simulink model "WindTunnelControl"  (R2023b)
settings: Solver=FixedStepDiscrete  StartTime=0.0  StopTime=Config.simulationTime  FixedStep=Config.tStep  RelTol=1e-3
InitFcn:
  | cd(fileparts(which(bdroot)));
  | initWindTunnelControl;
  | 
  | %% Try to edit the GUI (the user may have already closed it)
  | try
  | 
  |     %% Update Start Button
  |     set(sl_synch_handles.startButton,'Backgroundcolor',[0.0,1.0,0.0]);
  |     set(sl_synch_handles.startButton,'Enable','on');
  | end
StartFcn:
  | %% Try to edit the GUI (the user may have already closed it)
  | try
  | 
  |     %% Update Start Button
  |     set(sl_synch_handles.startButton,'Backgroundcolor',[0.8,0.8,0.8]);
  |     set(sl_synch_handles.startButton,'Enable','off');
  | 
  |     %% Update Compile Button
  |     set(sl_synch_handles.compileButton,'Backgroundcolor',[0.8,0.8,0.8]);
  |     set(sl_synch_handles.compileButton,'Enable','off');
  | 
  |     %% Update Exit Button
  |     set(sl_synch_handles.exitButton,'Backgroundcolor',[0.8,0.8,0.8]);
  |     set(sl_synch_handles.exitButton,'Enable','off');
  | end
StopFcn:
  | cd(fileparts(which(bdroot)));
  | stopWindTunnelControl;
  | 
  | %% Try to edit the GUI (the user may have already closed it)
  | try
  | 
  |     %% Update Start Button
  |     if get(sl_synch_handles.checkbox_recompile, 'Value')
  |         set(sl_synch_handles.startButton,'Backgroundcolor',[0.0,1.0,0.0]);
  |         set(sl_synch_handles.startButton,'Enable','on');
  |     end
  | 
  |     %% Update Compile Button
  |     set(sl_synch_handles.compileButton,'Backgroundcolor',[1.0,0.6,0.0]);
  |     set(sl_synch_handles.compileButton,'Enable','on');
  | 
  |     %% Update Exit Button
  |     set(sl_synch_handles.exitButton,'Backgroundcolor',[0.0,1.0,1.0]);
  |     set(sl_synch_handles.exitButton,'Enable','on');
  | end
undefined symbols (not defined in the file or in its folder): Config
libraries: dspsigattribs x44, WBToolboxLibrary x37, Get_System_State x1, Dynamics_and_Kinematics x1
CloseFcn:
  | %% Try to close the GUI (the user might have already closed it)
  | try
  | 
  |     close(simulinkStaticGUI)
  | end
settings Model: NumberOfSteps=50  Creator=gnava  LastModifiedBy=icub
settings SolverCC: AlgebraicLoopSolver=TrustRegion
settings DataIOCC: ReturnWorkspaceOutputs=off
settings OptimizationCC: BlockReduction=off  DefaultParameterBehavior=Inlined  BufferReuse=off  ReuseModelBlockBuffer=off
settings DebuggingCC: UnconnectedInputMsg=warning  UnconnectedOutputMsg=warning  UnconnectedLineMsg=warning  ArithmeticOperatorsInVariantConditions=warning
settings ModelReferenceCC: EnableRefExpFcnMdlSchedulingChecks=on
settings SFSimCC: SimUseLocalCustomCode=off  CustomCodeUndefinedFunction=UseInterfaceOnly
settings RTWCC: RTWUseLocalCustomCode=off  DLArmComputeVersion=19.05

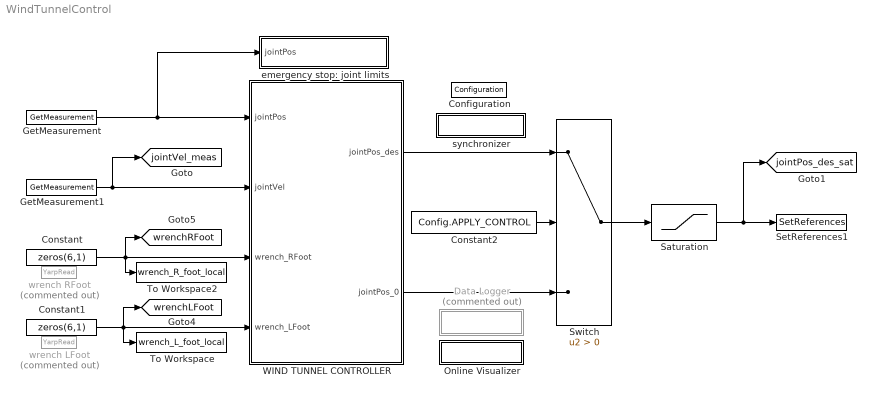
== system WindTunnelControl ==
  Configuration : WBToolboxLibrary/Utilities/Configuration  ConfigSource=Workspace  ConfigObject='WBTConfigRobot'
      settings: SourceProductName=WholeBodyToolbox
  Constant : Constant  Value=zeros(6,1)
  Constant1 : Constant  Value=zeros(6,1)
  Constant2 : Constant  Value=Config.APPLY_CONTROL  VectorParams1D=off  SampleTime=-1
  Data Logger : Subsystem  Commented=on
      mask Display: disp('DATA LOGGER')
  GetMeasurement : WBToolboxLibrary/States/GetMeasurement  measuredType=Joints Position
      settings: SourceProductName=WholeBodyToolbox
  GetMeasurement1 : WBToolboxLibrary/States/GetMeasurement  measuredType=Joints Velocity
      settings: SourceProductName=WholeBodyToolbox
  Online Visualizer : Subsystem
      mask Display: disp('VISUALIZER')
  Saturation : Saturate  UpperLimit=Config.sat.jointPositionLimits(:,2)  LowerLimit=Config.sat.jointPositionLimits(:,1)
  SetReferences1 : WBToolboxLibrary/Actuators/SetReferences  controlType=Position Direct  refSpeed=10*(pi/180)  refAcceleration=1000000*(pi/180)
      settings: SourceProductName=WholeBodyToolbox
  Switch : Switch  Criteria=u2 > Threshold  SaturateOnIntegerOverflow=off  InputSameDT=off
  To Workspace : ToWorkspace  VariableName=wrench_L_foot_local  SaveFormat=Structure With Time  SampleTime=-1
  To Workspace2 : ToWorkspace  VariableName=wrench_R_foot_local  SaveFormat=Structure With Time  SampleTime=-1
  WIND TUNNEL CONTROLLER : Subsystem
  emergency stop: joint limits : Subsystem
      mask Display: disp('EMERGENCY STOP')
  synchronizer : Subsystem
      mask Display: disp('SYNCHRONIZER')
  wrench LFoot : WBToolboxLibrary/Utilities/YarpRead  Commented=on  portName=Ports.WRENCH_LEFT_FOOT  signalSize=6  timeout=0.5  blocking=off  timestamp=off  autoconnect=on  errorOnConnection=on
      settings: SourceProductName=WholeBodyToolbox
  wrench RFoot : WBToolboxLibrary/Utilities/YarpRead  Commented=on  portName=Ports.WRENCH_RIGHT_FOOT  signalSize=6  timeout=0.5  blocking=off  timestamp=off  autoconnect=on  errorOnConnection=on
      settings: SourceProductName=WholeBodyToolbox
  tag scope: jointPos_des_sat=global, jointVel_meas=global, wrenchLFoot=global, wrenchRFoot=global
  wires:
  GetMeasurement1/1 -> [jointVel_meas], WIND TUNNEL CONTROLLER/2(jointVel)
  GetMeasurement/1 -> emergency stop: joint limits/1(jointPos), WIND TUNNEL CONTROLLER/1(jointPos)
  Constant2/1 -> Switch/2
  WIND TUNNEL CONTROLLER/1(jointPos_des) -> Switch/1
  Switch/1 -> Saturation/1
  WIND TUNNEL CONTROLLER/2(jointPos_0) -> Switch/3
  Saturation/1 -> [jointPos_des_sat], SetReferences1/1
  Constant1/1 -> [wrenchLFoot], To Workspace/1, WIND TUNNEL CONTROLLER/4(wrench_LFoot)
  Constant/1 -> To Workspace2/1, [wrenchRFoot], WIND TUNNEL CONTROLLER/3(wrench_RFoot)

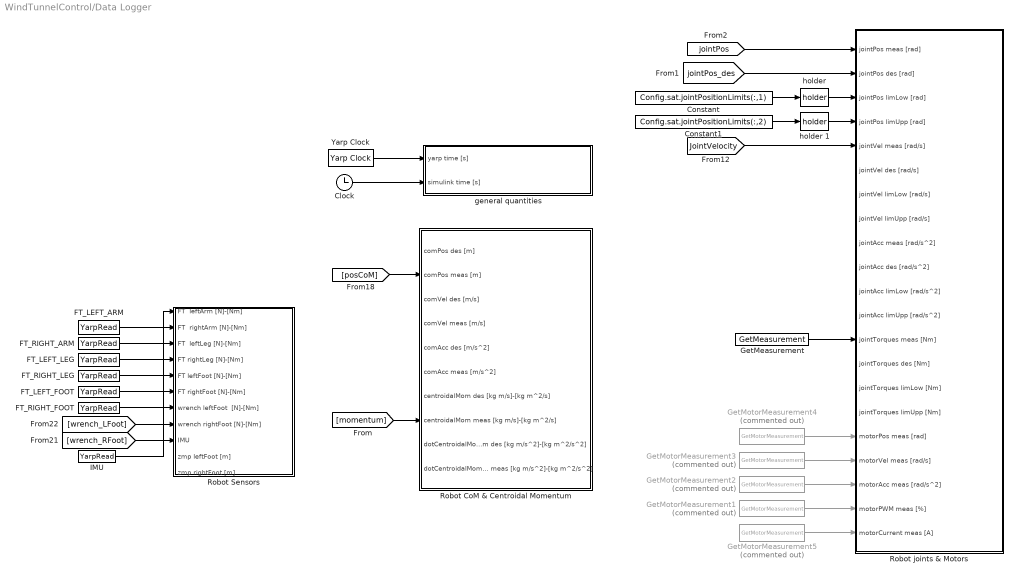
== system WindTunnelControl/Data Logger ==
  Clock : Clock
  Constant : Constant  Value=Config.sat.jointPositionLimits(:,1)
  Constant1 : Constant  Value=Config.sat.jointPositionLimits(:,2)
  FT_LEFT_ARM : WBToolboxLibrary/Utilities/YarpRead  portName=Ports.FT_LEFT_ARM  signalSize=6  timeout=0.5  blocking=off  timestamp=off  autoconnect=on  errorOnConnection=on
      settings: SourceProductName=WholeBodyToolbox
  FT_LEFT_FOOT : WBToolboxLibrary/Utilities/YarpRead  portName=Ports.FT_LEFT_FOOT  signalSize=6  timeout=0.5  blocking=off  timestamp=off  autoconnect=on  errorOnConnection=on
      settings: SourceProductName=WholeBodyToolbox
  FT_LEFT_LEG : WBToolboxLibrary/Utilities/YarpRead  portName=Ports.FT_LEFT_LEG  signalSize=6  timeout=0.5  blocking=off  timestamp=off  autoconnect=on  errorOnConnection=on
      settings: SourceProductName=WholeBodyToolbox
  FT_RIGHT_ARM : WBToolboxLibrary/Utilities/YarpRead  portName=Ports.FT_RIGHT_ARM  signalSize=6  timeout=0.5  blocking=off  timestamp=off  autoconnect=on  errorOnConnection=on
      settings: SourceProductName=WholeBodyToolbox
  FT_RIGHT_FOOT : WBToolboxLibrary/Utilities/YarpRead  portName=Ports.FT_RIGHT_FOOT  signalSize=6  timeout=0.5  blocking=off  timestamp=off  autoconnect=on  errorOnConnection=on
      settings: SourceProductName=WholeBodyToolbox
  FT_RIGHT_LEG : WBToolboxLibrary/Utilities/YarpRead  portName=Ports.FT_RIGHT_LEG  signalSize=6  timeout=0.5  blocking=off  timestamp=off  autoconnect=on  errorOnConnection=on
      settings: SourceProductName=WholeBodyToolbox
  GetMeasurement : WBToolboxLibrary/States/GetMeasurement  measuredType=Joints Torque
      settings: SourceProductName=WholeBodyToolbox
  GetMotorMeasurement1 : WBToolboxLibrary/States/GetMotorMeasurement  Commented=on  measuredType=Motor PWM
      settings: SourceProductName=WholeBodyToolbox
  GetMotorMeasurement2 : WBToolboxLibrary/States/GetMotorMeasurement  Commented=on  measuredType=Motor Acceleration
      settings: SourceProductName=WholeBodyToolbox
  GetMotorMeasurement3 : WBToolboxLibrary/States/GetMotorMeasurement  Commented=on  measuredType=Motor Velocity
      settings: SourceProductName=WholeBodyToolbox
  GetMotorMeasurement4 : WBToolboxLibrary/States/GetMotorMeasurement  Commented=on  measuredType=Motor Position
      settings: SourceProductName=WholeBodyToolbox
  GetMotorMeasurement5 : WBToolboxLibrary/States/GetMotorMeasurement  Commented=on  measuredType=Motor Current
      settings: SourceProductName=WholeBodyToolbox
  IMU : WBToolboxLibrary/Utilities/YarpRead  portName=Ports.IMU  signalSize=12  timeout=0.5  blocking=off  timestamp=off  autoconnect=on  errorOnConnection=on
      settings: SourceProductName=WholeBodyToolbox
  Robot CoM & Centroidal Momentum : Subsystem  AncestorBlock=data_dumper/Robot CoM & Centroidal Momentum
      settings: LibrarySourceBlock=data_dumper/Robot CoM & Centroidal Momentum
  Robot Sensors : Subsystem  AncestorBlock=data_dumper/Robot Sensors
      settings: LibrarySourceBlock=data_dumper/Robot Sensors
  Robot joints & Motors : Subsystem  AncestorBlock=data_dumper/Robot joints & Motors
      settings: LibrarySourceBlock=data_dumper/Robot joints & Motors
  Yarp Clock : WBToolboxLibrary/Utilities/Yarp Clock
      settings: SourceProductName=WholeBodyToolbox
  general quantities : Subsystem  AncestorBlock=data_dumper/general quantities
      settings: LibrarySourceBlock=data_dumper/general quantities
  "holder " : WBToolboxLibrary/Utilities/holder 
      settings: SourceProductName=WholeBodyToolbox
  holder 1 : WBToolboxLibrary/Utilities/holder 
      settings: SourceProductName=WholeBodyToolbox
  wires:
  Constant/1 -> "holder "/1
  Constant1/1 -> holder 1/1
  [JointVelocity] -> Robot joints & Motors/5(jointVel meas [rad/s])
  GetMeasurement/1 -> Robot joints & Motors/13("jointTorques meas [Nm] ")
  GetMotorMeasurement2/1 -> Robot joints & Motors/19(motorAcc meas [rad/s^2])
  GetMotorMeasurement3/1 -> Robot joints & Motors/18(motorVel meas [rad/s])
  GetMotorMeasurement4/1 -> Robot joints & Motors/17(motorPos meas [rad])
  Yarp Clock/1 -> general quantities/1(yarp time [s])
  Clock/1 -> general quantities/2(simulink time [s])
  [wrench_LFoot] -> Robot Sensors/7(wrench leftFoot  [N]-[Nm])
  [wrench_RFoot] -> Robot Sensors/8(wrench rightFoot [N]-[Nm])
  FT_LEFT_LEG/1 -> Robot Sensors/3(FT  leftLeg [N]-[Nm])
  FT_LEFT_ARM/1 -> Robot Sensors/1(FT  leftArm [N]-[Nm])
  FT_LEFT_FOOT/1 -> Robot Sensors/5(FT leftFoot [N]-[Nm])
  FT_RIGHT_ARM/1 -> Robot Sensors/2(FT  rightArm [N]-[Nm])
  FT_RIGHT_LEG/1 -> Robot Sensors/4(FT rightLeg [N]-[Nm])
  FT_RIGHT_FOOT/1 -> Robot Sensors/6(FT rightFoot [N]-[Nm])
  IMU/1 -> Robot Sensors/9(IMU)
  [posCoM] -> Robot CoM & Centroidal Momentum/2(comPos meas [m])
  [jointPos] -> Robot joints & Motors/1(jointPos meas [rad])
  [jointPos_des] -> Robot joints & Motors/2(jointPos des [rad])
  "holder "/1 -> Robot joints & Motors/3(jointPos limLow [rad])
  holder 1/1 -> Robot joints & Motors/4(jointPos limUpp [rad])
  [momentum] -> Robot CoM & Centroidal Momentum/8(centroidalMom meas [kg m/s]-[kg m^2/s])
  GetMotorMeasurement1/1 -> Robot joints & Motors/20("motorPWM meas [%] ")
  GetMotorMeasurement5/1 -> Robot joints & Motors/21(motorCurrent meas [A])

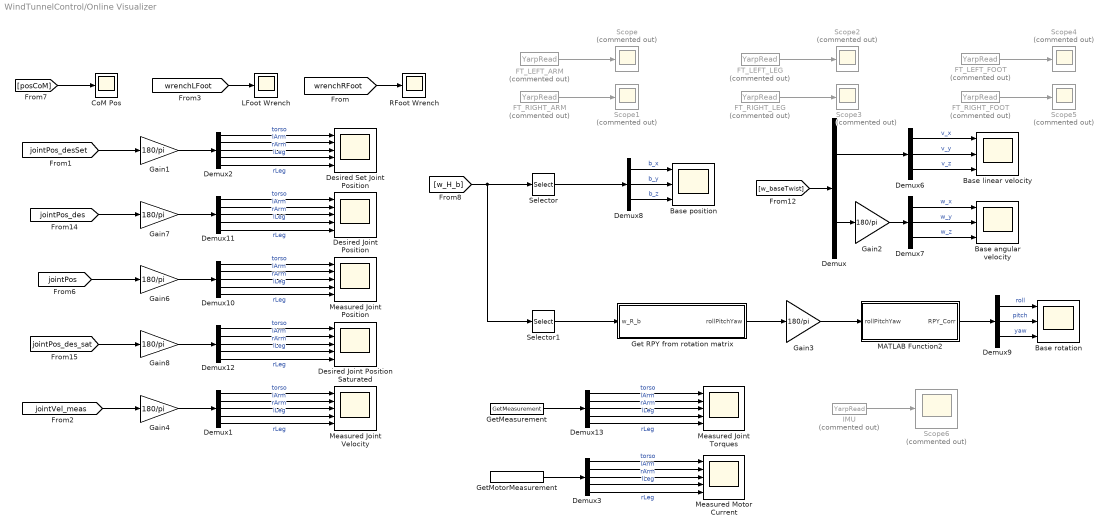
== system WindTunnelControl/Online Visualizer ==
  Base angular velocity : Scope  NumInputPorts=3
  Base linear velocity : Scope  NumInputPorts=3
  Base position : Scope  NumInputPorts=3
  Base rotation : Scope  NumInputPorts=3
  CoM Pos : Scope
  Demux : Demux  Outputs=2
  Demux{1..3,10..13} (7 alike) : Demux  Outputs=Config.numOfJointsForEachControlboard
  Demux{6..9} (4 alike) : Demux  Outputs=3
  Desired Joint Position : Scope  NumInputPorts=5
  Desired Joint Position Saturated : Scope  NumInputPorts=5
  Desired Set Joint Position : Scope  NumInputPorts=5
  FT_LEFT_ARM : WBToolboxLibrary/Utilities/YarpRead  Commented=on  portName=Ports.FT_LEFT_ARM  signalSize=6  timeout=0.5  blocking=off  timestamp=off  autoconnect=on  errorOnConnection=on
      settings: SourceProductName=WholeBodyToolbox
  FT_LEFT_FOOT : WBToolboxLibrary/Utilities/YarpRead  Commented=on  portName=Ports.FT_LEFT_FOOT  signalSize=6  timeout=0.5  blocking=off  timestamp=off  autoconnect=on  errorOnConnection=on
      settings: SourceProductName=WholeBodyToolbox
  FT_LEFT_LEG : WBToolboxLibrary/Utilities/YarpRead  Commented=on  portName=Ports.FT_LEFT_LEG  signalSize=6  timeout=0.5  blocking=off  timestamp=off  autoconnect=on  errorOnConnection=on
      settings: SourceProductName=WholeBodyToolbox
  FT_RIGHT_ARM : WBToolboxLibrary/Utilities/YarpRead  Commented=on  portName=Ports.FT_RIGHT_ARM  signalSize=6  timeout=0.5  blocking=off  timestamp=off  autoconnect=on  errorOnConnection=on
      settings: SourceProductName=WholeBodyToolbox
  FT_RIGHT_FOOT : WBToolboxLibrary/Utilities/YarpRead  Commented=on  portName=Ports.FT_RIGHT_FOOT  signalSize=6  timeout=0.5  blocking=off  timestamp=off  autoconnect=on  errorOnConnection=on
      settings: SourceProductName=WholeBodyToolbox
  FT_RIGHT_LEG : WBToolboxLibrary/Utilities/YarpRead  Commented=on  portName=Ports.FT_RIGHT_LEG  signalSize=6  timeout=0.5  blocking=off  timestamp=off  autoconnect=on  errorOnConnection=on
      settings: SourceProductName=WholeBodyToolbox
  Gain{1..4,6..8} (7 alike) : Gain  Gain=180/pi
  Get RPY from rotation matrix : MATLAB Function  TreatAsAtomicUnit=on
  GetMeasurement : WBToolboxLibrary/States/GetMeasurement  measuredType=Joints Torque
      settings: SourceProductName=WholeBodyToolbox
  GetMotorMeasurement : WBToolboxLibrary/States/GetMotorMeasurement  measuredType=Motor Current
      settings: SourceProductName=WholeBodyToolbox
  IMU : WBToolboxLibrary/Utilities/YarpRead  Commented=on  portName=Ports.IMU  signalSize=12  timeout=0.5  blocking=off  timestamp=off  autoconnect=on  errorOnConnection=on
      settings: SourceProductName=WholeBodyToolbox
  LFoot Wrench : Scope
  MATLAB Function2 : MATLAB Function  TreatAsAtomicUnit=on
  Measured Joint Position : Scope  NumInputPorts=5
  Measured Joint Torques : Scope  NumInputPorts=5
  Measured Joint Velocity : Scope  NumInputPorts=5
  Measured Motor Current : Scope  NumInputPorts=5
  RFoot Wrench : Scope
  Scope{,1..6} (7 alike) : Scope  Commented=on
  Selector : Selector  NumberOfDimensions=2  InputPortWidth=3  IndexOptions=Index vector (dialog),Index vector (dialog)  Indices=[1:3],4  OutputSizes=1,1
  Selector1 : Selector  NumberOfDimensions=2  InputPortWidth=3  IndexOptions=Index vector (dialog),Index vector (dialog)  Indices=[1:3],[1:3]  OutputSizes=1,1
  wires:
  Demux1/5 -> Measured Joint Velocity/5  "rLeg"
  Demux1/3 -> Measured Joint Velocity/3  "rArm"
  Demux1/1 -> Measured Joint Velocity/1  "torso"
  Demux1/4 -> Measured Joint Velocity/4  "lLeg"
  Gain4/1 -> Demux1/1
  [jointVel_meas] -> Gain4/1
  Demux1/2 -> Measured Joint Velocity/2  "lArm"
  [posCoM] -> CoM Pos/1
  [wrenchLFoot] -> LFoot Wrench/1
  [wrenchRFoot] -> RFoot Wrench/1
  Demux/2 -> Gain2/1
  Demux6/1 -> Base linear velocity/1  "v_x"
  Demux9/2 -> Base rotation/2  "pitch"
  Demux7/2 -> Base angular velocity/2  "w_y"
  [w_H_b] -> Selector1/1, Selector/1
  Demux6/2 -> Base linear velocity/2  "v_y"
  Gain3/1 -> MATLAB Function2/1(rollPitchYaw)
  Selector1/1 -> Get RPY from rotation matrix/1(w_R_b)
  Get RPY from rotation matrix/1(rollPitchYaw) -> Gain3/1
  Demux9/3 -> Base rotation/3  "yaw"
  Demux8/2 -> Base position/2  "b_y"
  Demux/1 -> Demux6/1
  Demux8/1 -> Base position/1  "b_x"
  Demux7/3 -> Base angular velocity/3  "w_z"
  MATLAB Function2/1(RPY_Corr) -> Demux9/1
  Gain2/1 -> Demux7/1
  Demux7/1 -> Base angular velocity/1  "w_x"
  Demux9/1 -> Base rotation/1  "roll"
  Demux6/3 -> Base linear velocity/3  "v_z"
  Selector/1 -> Demux8/1
  [w_baseTwist] -> Demux/1
  Demux8/3 -> Base position/3  "b_z"
  Demux10/4 -> Measured Joint Position/4  "lLeg"
  Demux10/2 -> Measured Joint Position/2  "lArm"
  [jointPos] -> Gain6/1
  Demux10/5 -> Measured Joint Position/5  "rLeg"
  Demux10/1 -> Measured Joint Position/1  "torso"
  Gain6/1 -> Demux10/1
  Demux10/3 -> Measured Joint Position/3  "rArm"
  Demux11/5 -> Desired Joint Position/5  "rLeg"
  Demux11/4 -> Desired Joint Position/4  "lLeg"
  Demux11/3 -> Desired Joint Position/3  "rArm"
  Gain7/1 -> Demux11/1
  Demux11/1 -> Desired Joint Position/1  "torso"
  [jointPos_des] -> Gain7/1
  Demux11/2 -> Desired Joint Position/2  "lArm"
  Demux12/2 -> Desired Joint Position Saturated/2  "lArm"
  Gain8/1 -> Demux12/1
  Demux12/3 -> Desired Joint Position Saturated/3  "rArm"
  Demux12/1 -> Desired Joint Position Saturated/1  "torso"
  [jointPos_des_sat] -> Gain8/1
  Demux12/4 -> Desired Joint Position Saturated/4  "lLeg"
  Demux12/5 -> Desired Joint Position Saturated/5  "rLeg"
  Demux13/2 -> Measured Joint Torques/2  "lArm"
  Demux13/3 -> Measured Joint Torques/3  "rArm"
  Demux13/1 -> Measured Joint Torques/1  "torso"
  GetMeasurement/1 -> Demux13/1
  Demux13/4 -> Measured Joint Torques/4  "lLeg"
  Demux13/5 -> Measured Joint Torques/5  "rLeg"
  Demux2/2 -> Desired Set Joint Position/2  "lArm"
  [jointPos_desSet] -> Gain1/1
  Gain1/1 -> Demux2/1
  Demux2/4 -> Desired Set Joint Position/4  "lLeg"
  Demux2/3 -> Desired Set Joint Position/3  "rArm"
  Demux2/1 -> Desired Set Joint Position/1  "torso"
  Demux2/5 -> Desired Set Joint Position/5  "rLeg"
  IMU/1 -> Scope6/1
  FT_LEFT_ARM/1 -> Scope/1
  FT_RIGHT_ARM/1 -> Scope1/1
  FT_RIGHT_LEG/1 -> Scope3/1
  FT_LEFT_LEG/1 -> Scope2/1
  FT_RIGHT_FOOT/1 -> Scope5/1
  FT_LEFT_FOOT/1 -> Scope4/1
  Demux3/3 -> Measured Motor Current/3  "rArm"
  GetMotorMeasurement/1 -> Demux3/1
  Demux3/4 -> Measured Motor Current/4  "lLeg"
  Demux3/5 -> Measured Motor Current/5  "rLeg"
  Demux3/2 -> Measured Motor Current/2  "lArm"
  Demux3/1 -> Measured Motor Current/1  "torso"

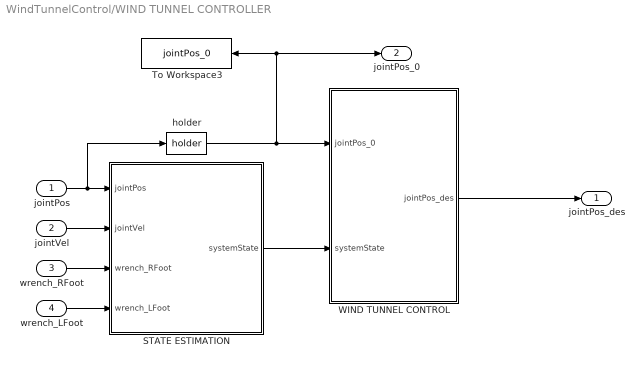
== system WindTunnelControl/WIND TUNNEL CONTROLLER ==
  jointPos : Inport
  jointVel : Inport  Port=2
  wrench_RFoot : Inport  Port=3
  wrench_LFoot : Inport  Port=4
  STATE ESTIMATION : Subsystem
  To Workspace3 : ToWorkspace  VariableName=jointPos_0  SaveFormat=Structure With Time  SampleTime=-1
  WIND TUNNEL CONTROL : Subsystem
  "holder " : WBToolboxLibrary/Utilities/holder 
      settings: SourceProductName=WholeBodyToolbox
  jointPos_des : Outport  VectorParamsAs1DForOutWhenUnconnected=off
  jointPos_0 : Outport  Port=2  VectorParamsAs1DForOutWhenUnconnected=off
  wires:
  WIND TUNNEL CONTROL/1(jointPos_des) -> jointPos_des/1
  jointPos/1 -> "holder "/1, STATE ESTIMATION/1(jointPos)
  jointVel/1 -> STATE ESTIMATION/2(jointVel)
  STATE ESTIMATION/1(systemState) -> WIND TUNNEL CONTROL/2(systemState)
  wrench_RFoot/1 -> STATE ESTIMATION/3(wrench_RFoot)
  wrench_LFoot/1 -> STATE ESTIMATION/4(wrench_LFoot)
  "holder "/1 -> jointPos_0/1, To Workspace3/1, WIND TUNNEL CONTROL/1(jointPos_0)

== system WindTunnelControl/emergency stop: joint limits ==
  jointPos : Inport
  ON_GAZEBO 1 : Constant  Value=Config.EMERGENCY_STOP_WITH_JOINTS_LIMITS
  ON_GAZEBO 2 : Constant  Value=Config.EMERGENCY_STOP_WITH_ENCODER_SPIKES
  STOP IF JOINTS HIT THE LIMITS : Subsystem
  STOP IF THERE ARE SPIKES IN THE ENCODERS : Subsystem
  wires:
  ON_GAZEBO 1/1 -> STOP IF JOINTS HIT THE LIMITS/Enable
  jointPos/1 -> STOP IF THERE ARE SPIKES IN THE ENCODERS/1(jointPos), STOP IF JOINTS HIT THE LIMITS/1(jointPos)
  ON_GAZEBO 2/1 -> STOP IF THERE ARE SPIKES IN THE ENCODERS/Enable

== system WindTunnelControl/synchronizer ==
  GAZEBO_SYNCHRONIZER : Subsystem
  Logical Operator : Logic  Operator=NOT  AllPortsSameDT=off  OutDataTypeStr=boolean
  "ON_GAZEBO " : Constant  Value=Config.ON_GAZEBO
  REAL_TIME_SYNC : Subsystem
  wires:
  Logical Operator/1 -> REAL_TIME_SYNC/Enable
  "ON_GAZEBO "/1 -> GAZEBO_SYNCHRONIZER/Enable, Logical Operator/1

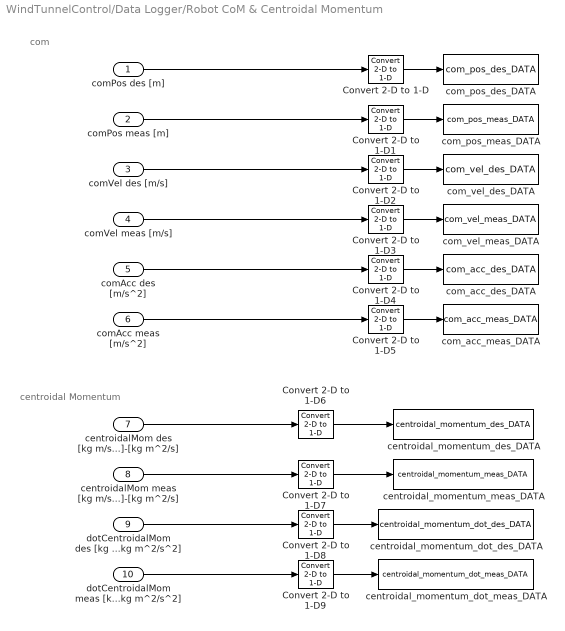
== system WindTunnelControl/Data Logger/Robot CoM & Centroidal Momentum ==
  note: centroidal Momentum
  note: com
  comPos des [m] : Inport
  comPos meas [m] : Inport  Port=2
  comVel des [m/s] : Inport  Port=3
  comVel meas [m/s] : Inport  Port=4
  comAcc des [m/s^2] : Inport  Port=5
  comAcc meas [m/s^2] : Inport  Port=6
  centroidalMom des [kg m/s]-[kg m^2/s] : Inport  Port=7
  centroidalMom meas [kg m/s]-[kg m^2/s] : Inport  Port=8
  dotCentroidalMom des [kg m/s^2]-[kg m^2/s^2] : Inport  Port=9
  dotCentroidalMom meas [kg m/s^2]-[kg m^2/s^2] : Inport  Port=10
  Convert 2-D to 1-D{,1..9} (10 alike) : dspsigattribs/Convert 2-D to 1-D
  centroidal_momentum_des_DATA : ToWorkspace  VariableName=centroidal_momentum_des_DATA  SaveFormat=Structure With Time  SampleTime=-1
  centroidal_momentum_dot_des_DATA : ToWorkspace  VariableName=centroidal_momentum_dot_des_DATA  SaveFormat=Structure With Time  SampleTime=-1
  centroidal_momentum_dot_meas_DATA : ToWorkspace  VariableName=centroidal_momentum_dot_meas_DATA  SaveFormat=Structure With Time  SampleTime=-1
  centroidal_momentum_meas_DATA : ToWorkspace  VariableName=centroidal_momentum_meas_DATA  SaveFormat=Structure With Time  SampleTime=-1
  com_acc_des_DATA : ToWorkspace  VariableName=com_acc_des_DATA  SaveFormat=Structure With Time  SampleTime=-1
  com_acc_meas_DATA : ToWorkspace  VariableName=com_acc_meas_DATA  SaveFormat=Structure With Time  SampleTime=-1
  com_pos_des_DATA : ToWorkspace  VariableName=com_pos_des_DATA  SaveFormat=Structure With Time  SampleTime=-1
  com_pos_meas_DATA : ToWorkspace  VariableName=com_pos_meas_DATA  SaveFormat=Structure With Time  SampleTime=-1
  com_vel_des_DATA : ToWorkspace  VariableName=com_vel_des_DATA  SaveFormat=Structure With Time  SampleTime=-1
  com_vel_meas_DATA : ToWorkspace  VariableName=com_vel_meas_DATA  SaveFormat=Structure With Time  SampleTime=-1
  wires:
  Convert 2-D to 1-D9/1 -> centroidal_momentum_dot_meas_DATA/1
  Convert 2-D to 1-D8/1 -> centroidal_momentum_dot_des_DATA/1
  Convert 2-D to 1-D7/1 -> centroidal_momentum_meas_DATA/1
  Convert 2-D to 1-D6/1 -> centroidal_momentum_des_DATA/1
  Convert 2-D to 1-D5/1 -> com_acc_meas_DATA/1
  Convert 2-D to 1-D4/1 -> com_acc_des_DATA/1
  Convert 2-D to 1-D3/1 -> com_vel_meas_DATA/1
  Convert 2-D to 1-D2/1 -> com_vel_des_DATA/1
  Convert 2-D to 1-D1/1 -> com_pos_meas_DATA/1
  Convert 2-D to 1-D/1 -> com_pos_des_DATA/1
  dotCentroidalMom meas [kg m/s^2]-[kg m^2/s^2]/1 -> Convert 2-D to 1-D9/1
  centroidalMom des [kg m/s]-[kg m^2/s]/1 -> Convert 2-D to 1-D6/1
  centroidalMom meas [kg m/s]-[kg m^2/s]/1 -> Convert 2-D to 1-D7/1
  dotCentroidalMom des [kg m/s^2]-[kg m^2/s^2]/1 -> Convert 2-D to 1-D8/1
  comVel meas [m/s]/1 -> Convert 2-D to 1-D3/1
  comPos meas [m]/1 -> Convert 2-D to 1-D1/1
  comAcc meas [m/s^2]/1 -> Convert 2-D to 1-D5/1
  comPos des [m]/1 -> Convert 2-D to 1-D/1
  comAcc des [m/s^2]/1 -> Convert 2-D to 1-D4/1
  comVel des [m/s]/1 -> Convert 2-D to 1-D2/1

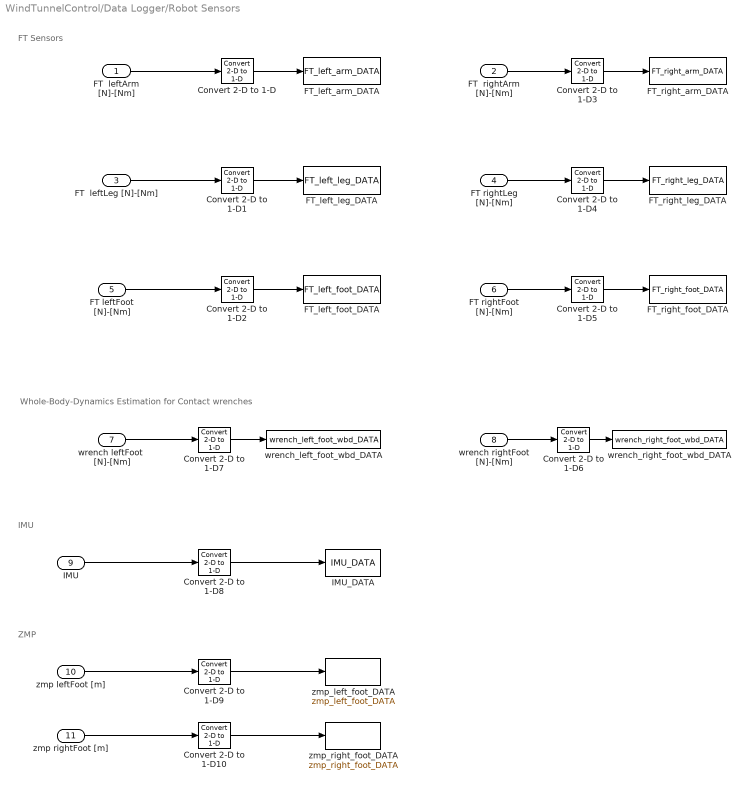
== system WindTunnelControl/Data Logger/Robot Sensors ==
  note: ZMP
  note: IMU
  note: FT Sensors
  note: Whole-Body-Dynamics Estimation for Contact wrenches
  FT  leftArm [N]-[Nm] : Inport
  FT  rightArm [N]-[Nm] : Inport  Port=2
  FT  leftLeg [N]-[Nm] : Inport  Port=3
  FT rightLeg [N]-[Nm] : Inport  Port=4
  FT leftFoot [N]-[Nm] : Inport  Port=5
  FT rightFoot [N]-[Nm] : Inport  Port=6
  wrench leftFoot  [N]-[Nm] : Inport  Port=7
  wrench rightFoot [N]-[Nm] : Inport  Port=8
  IMU : Inport  Port=9
  zmp leftFoot [m] : Inport  Port=10
  zmp rightFoot [m] : Inport  Port=11
  Convert 2-D to 1-D{,1..10} (11 alike) : dspsigattribs/Convert 2-D to 1-D
  FT_left_arm_DATA : ToWorkspace  VariableName=FT_left_arm_DATA  SaveFormat=Structure With Time  SampleTime=-1
  FT_left_foot_DATA : ToWorkspace  VariableName=FT_left_foot_DATA  SaveFormat=Structure With Time  SampleTime=-1
  FT_left_leg_DATA : ToWorkspace  VariableName=FT_left_leg_DATA  SaveFormat=Structure With Time  SampleTime=-1
  FT_right_arm_DATA : ToWorkspace  VariableName=FT_right_arm_DATA  SaveFormat=Structure With Time  SampleTime=-1
  FT_right_foot_DATA : ToWorkspace  VariableName=FT_right_foot_DATA  SaveFormat=Structure With Time  SampleTime=-1
  FT_right_leg_DATA : ToWorkspace  VariableName=FT_right_leg_DATA  SaveFormat=Structure With Time  SampleTime=-1
  IMU_DATA : ToWorkspace  VariableName=IMU_DATA  SaveFormat=Structure With Time  SampleTime=-1
  wrench_left_foot_wbd_DATA : ToWorkspace  VariableName=wrench_left_foot_wbd_DATA  SaveFormat=Structure With Time  SampleTime=-1
  wrench_right_foot_wbd_DATA : ToWorkspace  VariableName=wrench_right_foot_wbd_DATA  SaveFormat=Structure With Time  SampleTime=-1
  zmp_left_foot_DATA : ToWorkspace  VariableName=zmp_left_foot_DATA  SaveFormat=Structure With Time  SampleTime=-1
  zmp_right_foot_DATA : ToWorkspace  VariableName=zmp_right_foot_DATA  SaveFormat=Structure With Time  SampleTime=-1
  wires:
  zmp rightFoot [m]/1 -> Convert 2-D to 1-D10/1
  Convert 2-D to 1-D10/1 -> zmp_right_foot_DATA/1
  zmp leftFoot [m]/1 -> Convert 2-D to 1-D9/1
  Convert 2-D to 1-D9/1 -> zmp_left_foot_DATA/1
  Convert 2-D to 1-D8/1 -> IMU_DATA/1
  Convert 2-D to 1-D7/1 -> wrench_left_foot_wbd_DATA/1
  Convert 2-D to 1-D6/1 -> wrench_right_foot_wbd_DATA/1
  Convert 2-D to 1-D5/1 -> FT_right_foot_DATA/1
  Convert 2-D to 1-D4/1 -> FT_right_leg_DATA/1
  Convert 2-D to 1-D3/1 -> FT_right_arm_DATA/1
  Convert 2-D to 1-D2/1 -> FT_left_foot_DATA/1
  Convert 2-D to 1-D1/1 -> FT_left_leg_DATA/1
  Convert 2-D to 1-D/1 -> FT_left_arm_DATA/1
  wrench rightFoot [N]-[Nm]/1 -> Convert 2-D to 1-D6/1
  wrench leftFoot  [N]-[Nm]/1 -> Convert 2-D to 1-D7/1
  IMU/1 -> Convert 2-D to 1-D8/1
  FT  leftLeg [N]-[Nm]/1 -> Convert 2-D to 1-D1/1
  FT leftFoot [N]-[Nm]/1 -> Convert 2-D to 1-D2/1
  FT rightFoot [N]-[Nm]/1 -> Convert 2-D to 1-D5/1
  FT rightLeg [N]-[Nm]/1 -> Convert 2-D to 1-D4/1
  FT  rightArm [N]-[Nm]/1 -> Convert 2-D to 1-D3/1
  FT  leftArm [N]-[Nm]/1 -> Convert 2-D to 1-D/1

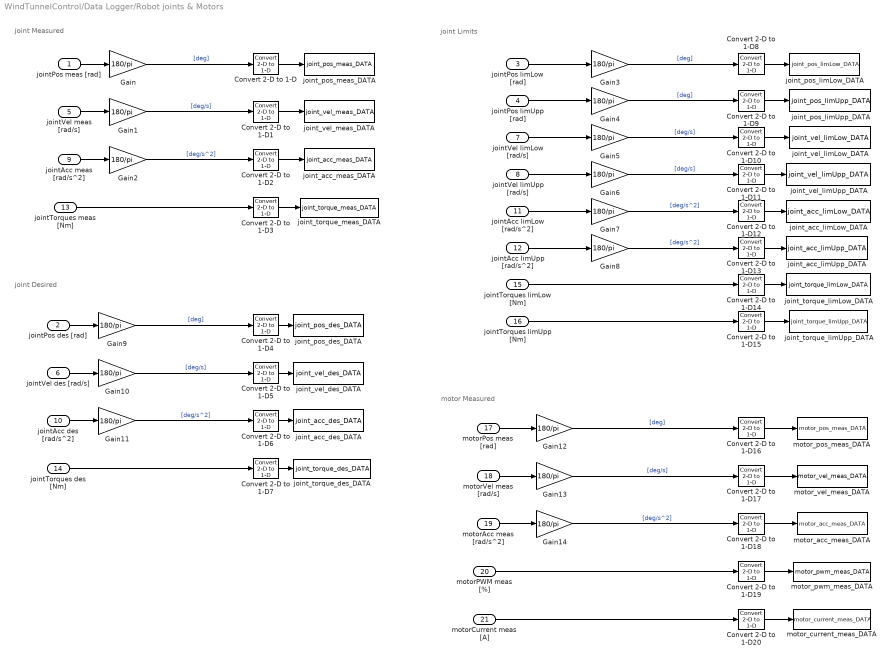
== system WindTunnelControl/Data Logger/Robot joints & Motors ==
  note: motor Measured
  note: joint Desired
  note: joint Measured
  note: joint Limits
  jointPos meas [rad] : Inport
  jointPos des [rad] : Inport  Port=2
  jointPos limLow [rad] : Inport  Port=3
  jointPos limUpp [rad] : Inport  Port=4
  jointVel meas [rad/s] : Inport  Port=5
  jointVel des [rad/s] : Inport  Port=6
  jointVel limLow [rad/s] : Inport  Port=7
  jointVel limUpp [rad/s] : Inport  Port=8
  jointAcc meas [rad/s^2] : Inport  Port=9
  jointAcc des [rad/s^2] : Inport  Port=10
  jointAcc limLow [rad/s^2] : Inport  Port=11
  jointAcc limUpp [rad/s^2] : Inport  Port=12
  "jointTorques meas [Nm] " : Inport  Port=13
  "jointTorques des [Nm] " : Inport  Port=14
  jointTorques limLow [Nm] : Inport  Port=15
  jointTorques limUpp [Nm] : Inport  Port=16
  motorPos meas [rad] : Inport  Port=17
  motorVel meas [rad/s] : Inport  Port=18
  motorAcc meas [rad/s^2] : Inport  Port=19
  "motorPWM meas [%] " : Inport  Port=20
  motorCurrent meas [A] : Inport  Port=21
  Convert 2-D to 1-D{,1..20} (21 alike) : dspsigattribs/Convert 2-D to 1-D
  Gain{,1..14} (15 alike) : Gain  Gain=180/pi
  joint_acc_des_DATA : ToWorkspace  VariableName=joint_acc_des_DATA  SaveFormat=Structure With Time  SampleTime=-1
  joint_acc_limLow_DATA : ToWorkspace  VariableName=joint_acc_limLow_DATA  SaveFormat=Structure With Time  SampleTime=-1
  joint_acc_limUpp_DATA : ToWorkspace  VariableName=joint_acc_limUpp_DATA  SaveFormat=Structure With Time  SampleTime=-1
  joint_acc_meas_DATA : ToWorkspace  VariableName=joint_acc_meas_DATA  SaveFormat=Structure With Time  SampleTime=-1
  joint_pos_des_DATA : ToWorkspace  VariableName=joint_pos_des_DATA  SaveFormat=Structure With Time  SampleTime=-1
  joint_pos_limLow_DATA : ToWorkspace  VariableName=joint_pos_limLow_DATA  SaveFormat=Structure With Time  SampleTime=-1
  joint_pos_limUpp_DATA : ToWorkspace  VariableName=joint_pos_limUpp_DATA  SaveFormat=Structure With Time  SampleTime=-1
  joint_pos_meas_DATA : ToWorkspace  VariableName=joint_pos_meas_DATA  SaveFormat=Structure With Time  SampleTime=-1
  joint_torque_des_DATA : ToWorkspace  VariableName=joint_torque_des_DATA  SaveFormat=Structure With Time  SampleTime=-1
  joint_torque_limLow_DATA : ToWorkspace  VariableName=joint_torque_limLow_DATA  SaveFormat=Structure With Time  SampleTime=-1
  joint_torque_limUpp_DATA : ToWorkspace  VariableName=joint_torque_limUpp_DATA  SaveFormat=Structure With Time  SampleTime=-1
  joint_torque_meas_DATA : ToWorkspace  VariableName=joint_torque_meas_DATA  SaveFormat=Structure With Time  SampleTime=-1
  joint_vel_des_DATA : ToWorkspace  VariableName=joint_vel_des_DATA  SaveFormat=Structure With Time  SampleTime=-1
  joint_vel_limLow_DATA : ToWorkspace  VariableName=joint_vel_limLow_DATA  SaveFormat=Structure With Time  SampleTime=-1
  joint_vel_limUpp_DATA : ToWorkspace  VariableName=joint_vel_limUpp_DATA  SaveFormat=Structure With Time  SampleTime=-1
  joint_vel_meas_DATA : ToWorkspace  VariableName=joint_vel_meas_DATA  SaveFormat=Structure With Time  SampleTime=-1
  motor_acc_meas_DATA : ToWorkspace  VariableName=motor_acc_meas_DATA  SaveFormat=Structure With Time  SampleTime=-1
  motor_current_meas_DATA : ToWorkspace  VariableName=motor_current_meas_DATA  SaveFormat=Structure With Time  SampleTime=-1
  motor_pos_meas_DATA : ToWorkspace  VariableName=motor_pos_meas_DATA  SaveFormat=Structure With Time  SampleTime=-1
  motor_pwm_meas_DATA : ToWorkspace  VariableName=motor_pwm_meas_DATA  SaveFormat=Structure With Time  SampleTime=-1
  motor_vel_meas_DATA : ToWorkspace  VariableName=motor_vel_meas_DATA  SaveFormat=Structure With Time  SampleTime=-1
  wires:
  Convert 2-D to 1-D20/1 -> motor_current_meas_DATA/1
  Convert 2-D to 1-D19/1 -> motor_pwm_meas_DATA/1
  Convert 2-D to 1-D18/1 -> motor_acc_meas_DATA/1
  Convert 2-D to 1-D17/1 -> motor_vel_meas_DATA/1
  Convert 2-D to 1-D16/1 -> motor_pos_meas_DATA/1
  Convert 2-D to 1-D15/1 -> joint_torque_limUpp_DATA/1
  Convert 2-D to 1-D14/1 -> joint_torque_limLow_DATA/1
  Convert 2-D to 1-D13/1 -> joint_acc_limUpp_DATA/1
  Convert 2-D to 1-D12/1 -> joint_acc_limLow_DATA/1
  Convert 2-D to 1-D11/1 -> joint_vel_limUpp_DATA/1
  Convert 2-D to 1-D10/1 -> joint_vel_limLow_DATA/1
  Convert 2-D to 1-D9/1 -> joint_pos_limUpp_DATA/1
  Convert 2-D to 1-D8/1 -> joint_pos_limLow_DATA/1
  Convert 2-D to 1-D7/1 -> joint_torque_des_DATA/1
  Convert 2-D to 1-D6/1 -> joint_acc_des_DATA/1
  Convert 2-D to 1-D5/1 -> joint_vel_des_DATA/1
  Convert 2-D to 1-D4/1 -> joint_pos_des_DATA/1
  Convert 2-D to 1-D3/1 -> joint_torque_meas_DATA/1
  Convert 2-D to 1-D2/1 -> joint_acc_meas_DATA/1
  Convert 2-D to 1-D1/1 -> joint_vel_meas_DATA/1
  Convert 2-D to 1-D/1 -> joint_pos_meas_DATA/1
  Gain13/1 -> Convert 2-D to 1-D17/1  "[deg/s]"
  motorAcc meas [rad/s^2]/1 -> Gain14/1
  "motorPWM meas [%] "/1 -> Convert 2-D to 1-D19/1
  motorVel meas [rad/s]/1 -> Gain13/1
  motorCurrent meas [A]/1 -> Convert 2-D to 1-D20/1
  Gain12/1 -> Convert 2-D to 1-D16/1  "[deg]"
  motorPos meas [rad]/1 -> Gain12/1
  Gain14/1 -> Convert 2-D to 1-D18/1  "[deg/s^2]"
  jointAcc des [rad/s^2]/1 -> Gain11/1
  Gain10/1 -> Convert 2-D to 1-D5/1  "[deg/s]"
  "jointTorques des [Nm] "/1 -> Convert 2-D to 1-D7/1
  Gain9/1 -> Convert 2-D to 1-D4/1  "[deg]"
  jointVel des [rad/s]/1 -> Gain10/1
  Gain11/1 -> Convert 2-D to 1-D6/1  "[deg/s^2]"
  jointPos des [rad]/1 -> Gain9/1
  jointTorques limUpp [Nm]/1 -> Convert 2-D to 1-D15/1
  jointTorques limLow [Nm]/1 -> Convert 2-D to 1-D14/1
  Gain8/1 -> Convert 2-D to 1-D13/1  "[deg/s^2]"
  Gain6/1 -> Convert 2-D to 1-D11/1  "[deg/s]"
  Gain7/1 -> Convert 2-D to 1-D12/1  "[deg/s^2]"
  Gain5/1 -> Convert 2-D to 1-D10/1  "[deg/s]"
  Gain4/1 -> Convert 2-D to 1-D9/1  "[deg]"
  Gain3/1 -> Convert 2-D to 1-D8/1  "[deg]"
  jointVel limUpp [rad/s]/1 -> Gain6/1
  jointAcc limLow [rad/s^2]/1 -> Gain7/1
  jointAcc limUpp [rad/s^2]/1 -> Gain8/1
  jointVel limLow [rad/s]/1 -> Gain5/1
  jointPos limUpp [rad]/1 -> Gain4/1
  jointPos limLow [rad]/1 -> Gain3/1
  "jointTorques meas [Nm] "/1 -> Convert 2-D to 1-D3/1
  Gain2/1 -> Convert 2-D to 1-D2/1  "[deg/s^2]"
  Gain1/1 -> Convert 2-D to 1-D1/1  "[deg/s]"
  jointAcc meas [rad/s^2]/1 -> Gain2/1
  jointVel meas [rad/s]/1 -> Gain1/1
  Gain/1 -> Convert 2-D to 1-D/1  "[deg]"
  jointPos meas [rad]/1 -> Gain/1

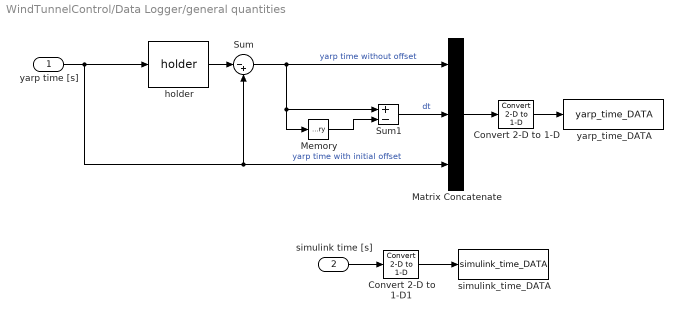
== system WindTunnelControl/Data Logger/general quantities ==
  yarp time [s] : Inport
  simulink time [s] : Inport  Port=2
  Convert 2-D to 1-D : dspsigattribs/Convert 2-D to 1-D
  Convert 2-D to 1-D1 : dspsigattribs/Convert 2-D to 1-D
  Matrix Concatenate : Concatenate  NumInputs=3
  Memory : Memory
  Sum : Sum  Inputs=|-+
  Sum1 : Sum  Inputs=+-
  "holder " : WBToolboxLibrary/Utilities/holder 
      settings: SourceProductName=WholeBodyToolbox
  simulink_time_DATA : ToWorkspace  VariableName=simulink_time_DATA  SaveFormat=Structure With Time  SampleTime=-1
  yarp_time_DATA : ToWorkspace  VariableName=yarp_time_DATA  SaveFormat=Structure With Time  SampleTime=-1
  wires:
  Convert 2-D to 1-D1/1 -> simulink_time_DATA/1
  Convert 2-D to 1-D/1 -> yarp_time_DATA/1
  Memory/1 -> Sum1/2
  Sum1/1 -> Matrix Concatenate/2  "dt"
  "holder "/1 -> Sum/1
  Sum/1 -> Sum1/1, Memory/1, Matrix Concatenate/1  "yarp time without offset"
  Matrix Concatenate/1 -> Convert 2-D to 1-D/1
  simulink time [s]/1 -> Convert 2-D to 1-D1/1
  yarp time [s]/1 -> "holder "/1, Matrix Concatenate/3, Sum/2  "yarp time with initial offset"

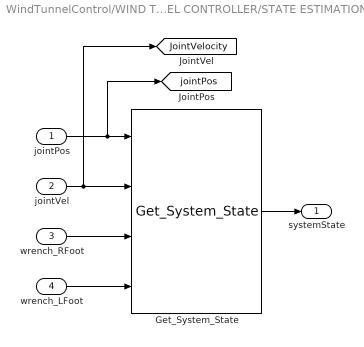
== system WindTunnelControl/WIND TUNNEL CONTROLLER/STATE ESTIMATION ==
  jointPos : Inport
  jointVel : Inport  Port=2
  wrench_RFoot : Inport  Port=3
  wrench_LFoot : Inport  Port=4
  Get_System_State : Get_System_State/Get_System_State  SystemSampleTime=-1  VariantActivationTime=update diagram  AllowFlexibleInterface=on  Latency=0  AutoFrameSizeCalculation=off
  systemState : Outport
  tag scope: JointVelocity=global, jointPos=global
  wires:
  Get_System_State/1 -> systemState/1
  jointPos/1 -> Get_System_State/1, [jointPos]
  jointVel/1 -> Get_System_State/2, [JointVelocity]
  wrench_LFoot/1 -> Get_System_State/4
  wrench_RFoot/1 -> Get_System_State/3

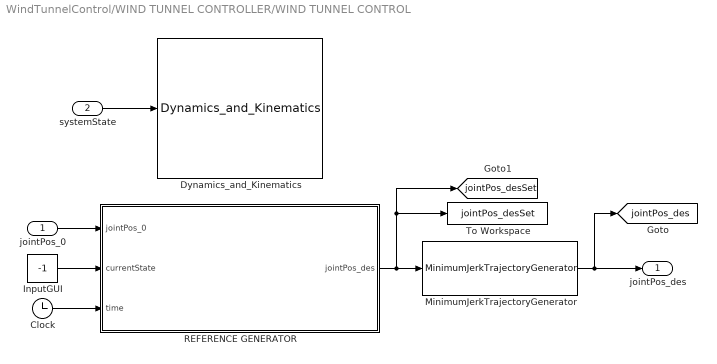
== system WindTunnelControl/WIND TUNNEL CONTROLLER/WIND TUNNEL CONTROL ==
  jointPos_0 : Inport
  systemState : Inport  Port=2
  Clock : Clock
  Dynamics_and_Kinematics : Dynamics_and_Kinematics/Dynamics_and_Kinematics  SystemSampleTime=-1  VariantActivationTime=update diagram  AllowFlexibleInterface=on  Latency=0  AutoFrameSizeCalculation=off
  InputGUI : Constant  Value=-1  SampleTime=-1
  MinimumJerkTrajectoryGenerator : WBToolboxLibrary/Utilities/MinimumJerkTrajectoryGenerator  externalSettlingTime=off  settlingTime=Config.tSettle  sampleTime=Config.tStep  resetOnSettlingTime=off  firstDerivatives=off  secondDerivatives=off  explicitInitialValue=off
      settings: SourceProductName=WholeBodyToolbox
  REFERENCE GENERATOR : MATLAB Function  TreatAsAtomicUnit=on
  To Workspace : ToWorkspace  VariableName=jointPos_desSet  SaveFormat=Structure With Time  SampleTime=-1
  jointPos_des : Outport  VectorParamsAs1DForOutWhenUnconnected=off
  tag scope: jointPos_des=global, jointPos_desSet=global
  wires:
  MinimumJerkTrajectoryGenerator/1 -> jointPos_des/1, [jointPos_des]
  systemState/1 -> Dynamics_and_Kinematics/1
  REFERENCE GENERATOR/1(jointPos_des) -> [jointPos_desSet], To Workspace/1, MinimumJerkTrajectoryGenerator/1
  jointPos_0/1 -> REFERENCE GENERATOR/1(jointPos_0)
  InputGUI/1 -> REFERENCE GENERATOR/2(currentState)
  Clock/1 -> REFERENCE GENERATOR/3(time)

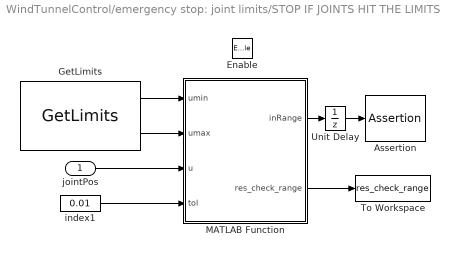
== system WindTunnelControl/emergency stop: joint limits/STOP IF JOINTS HIT THE LIMITS ==
  jointPos : Inport
  Enable : EnablePort
  Assertion : Assertion
  GetLimits : WBToolboxLibrary/States/GetLimits  limitsSource=ControlBoard  limitsType=Position
      settings: SourceProductName=WholeBodyToolbox
  MATLAB Function : MATLAB Function  TreatAsAtomicUnit=on
  To Workspace : ToWorkspace  VariableName=res_check_range  SaveFormat=Structure With Time  SampleTime=Config.tStep
  Unit Delay : UnitDelay  InitialCondition=1  SampleTime=Config.tStep  HasFrameUpgradeWarning=on
  index1 : Constant  Value=0.01  VectorParams1D=off
  wires:
  jointPos/1 -> MATLAB Function/3(u)
  MATLAB Function/1(inRange) -> Unit Delay/1
  index1/1 -> MATLAB Function/4(tol)
  MATLAB Function/2(res_check_range) -> To Workspace/1
  Unit Delay/1 -> Assertion/1
  GetLimits/1 -> MATLAB Function/1(umin)
  GetLimits/2 -> MATLAB Function/2(umax)

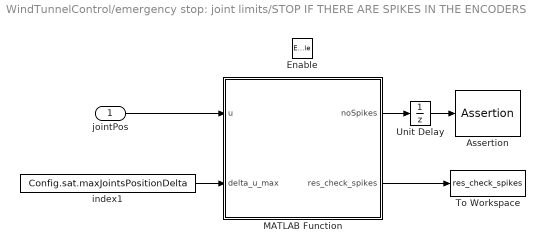
== system WindTunnelControl/emergency stop: joint limits/STOP IF THERE ARE SPIKES IN THE ENCODERS ==
  jointPos : Inport
  Enable : EnablePort
  Assertion : Assertion
  MATLAB Function : MATLAB Function  TreatAsAtomicUnit=on
  To Workspace : ToWorkspace  VariableName=res_check_spikes  SaveFormat=Structure With Time  SampleTime=Config.tStep
  Unit Delay : UnitDelay  InitialCondition=1  SampleTime=Config.tStep  HasFrameUpgradeWarning=on
  index1 : Constant  Value=Config.sat.maxJointsPositionDelta  VectorParams1D=off
  wires:
  jointPos/1 -> MATLAB Function/1(u)
  MATLAB Function/1(noSpikes) -> Unit Delay/1
  index1/1 -> MATLAB Function/2(delta_u_max)
  MATLAB Function/2(res_check_spikes) -> To Workspace/1
  Unit Delay/1 -> Assertion/1

== system WindTunnelControl/synchronizer/GAZEBO_SYNCHRONIZER ==
  Enable : EnablePort
  Simulator Synchronizer : WBToolboxLibrary/Utilities/Simulator Synchronizer  period=Config.tStep  serverPortName='/clock/rpc'  clientPortName='/WBT_synchronizer/rpc:o'
      settings: SourceProductName=WholeBodyToolbox

== system WindTunnelControl/synchronizer/REAL_TIME_SYNC ==
  Enable : EnablePort
  Real Time Synchronizer : WBToolboxLibrary/Utilities/Real Time Synchronizer  period=Config.tStep
      settings: SourceProductName=WholeBodyToolbox

== matlab function WindTunnelControl/emergency stop: joint limits/STOP IF THERE ARE SPIKES IN THE ENCODERS/MATLAB Function ==
  data: u input; delta_u_max input; noSpikes output; res_check_spikes output
function [noSpikes, res_check_spikes] = checkInputSpikesFCN(u, delta_u_max)

     [noSpikes, res_check_spikes] = wbc.checkInputSpikes(u, delta_u_max);
end

== matlab function WindTunnelControl/emergency stop: joint limits/STOP IF JOINTS HIT THE LIMITS/MATLAB Function ==
  data: umin input; umax input; u input; inRange output; tol input; res_check_range output
function [inRange, res_check_range] = checkInputRangeFCN(umin, umax, u, tol)

     [inRange, res_check_range] = wbc.checkInputRange(umin, umax, u, tol);
end

== matlab function WindTunnelControl/Online Visualizer/Get RPY from rotation matrix ==
  data: w_R_b input; rollPitchYaw output
function rollPitchYaw = rollPitchYawFromRotationFCN(w_R_b)

rollPitchYaw = wbc.rollPitchYawFromRotation(w_R_b);

end

== matlab function WindTunnelControl/Online Visualizer/MATLAB Function2 ==
  data: RPY_Corr output; rollPitchYaw input
function RPY_Corr = correctYawAngleFCN(rollPitchYaw)

    RPY_Corr = correctYawAngle(rollPitchYaw);

end

== matlab function WindTunnelControl/WIND TUNNEL CONTROLLER/WIND TUNNEL CONTROL/REFERENCE GENERATOR ==
  data: jointPos_0 input; currentState input; jointPos_des output; Config parameter; time input
function jointPos_des  = windTunnelReferenceGeneratorFCN(jointPos_0, currentState, Config, time)
 
    [jointPos_des] = windTunnelReferenceGenerator(jointPos_0, currentState, Config, time);
end
